simulink model "fusor_dynamical_model"  (R2024b)
settings: Solver=VariableStepAuto  StartTime=0.0  StopTime=10.0  RelTol=1e-3
settings Model: Creator=leone  LastModifiedBy=leone

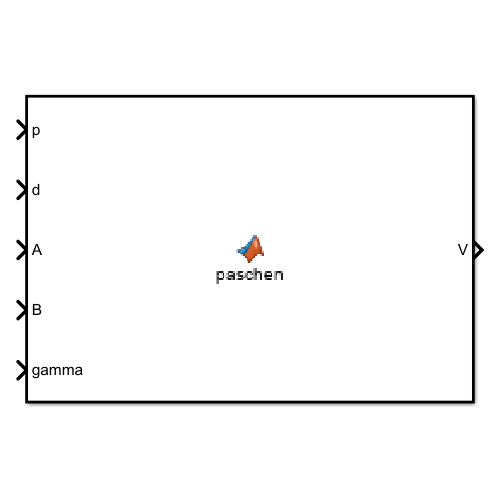
[thumbnail: Simulink's stored preview of the top-level diagram]
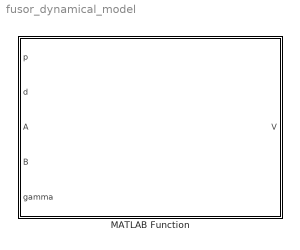
== system fusor_dynamical_model ==
  MATLAB Function : MATLAB Function  TreatAsAtomicUnit=on

== matlab function fusor_dynamical_model/MATLAB Function ==
  data: p input; V output; d input; A input; B input; gamma input
function V = paschen(p, d, A, B, gamma)
    V = (B .* p .* d) ./ (log(A .* p .* d) - log(log(1 + 1/gamma)));
end
